simulink model "MPC_Tracking_2020a"  (R2020a)
settings: Solver=VariableStepAuto  StartTime=0.0  StopTime=40  RelTol=1e-3
PostLoadFcn:
  | run('MPC_Tracking_init.m')
  | 
values from neighbouring files (symbols this model uses):
  A = [-1 0; 1 0]    [MPC_Tracking_init.m]
  B = [1;0]    [MPC_Tracking_init.m]
  C = [0,1]    [MPC_Tracking_init.m]
  F = 2*[K_'*Q_*S_; -T_*S_]'    [MPC_Tracking_init.m]
  G = [G;kron(eye(N),-eye(1))]    [MPC_Tracking_init.m]
  H = S_'*Q_*S_ + R_    [MPC_Tracking_init.m]
  N = 10    [MPC_Tracking_init.m]
  S = [zeros(2*N,3)]    [MPC_Tracking_init.m]
  Ts = 1    [MPC_Tracking_init.m]
  W = [delta_umax*ones(N,1);-delta_umin*ones(N,1)]    [MPC_Tracking_init.m]
  x_0 = [8 -5]'    [MPC_Tracking_init.m]
settings Model: Creator=hassan  LastModifiedBy=hassan

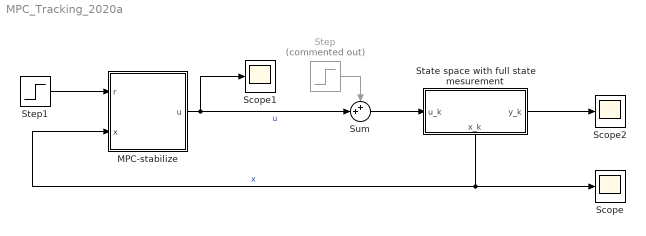
== system MPC_Tracking_2020a ==
  MPC-stabilize : Subsystem
  Scope : Scope
  Scope1 : Scope
  Scope2 : Scope
  State space with full state mesurement : Subsystem
      settings: PortSchema="{\"entries\":[{\"content\":{\"sides\":[{\"content\":{\"connectorIds\":[\"In1\"]},\"type\":\"ConnectorPlacement.EquallySpacedRectSide\",\"uuid\":\"af8233aa-8abb-4886-bf43-cd1df4b87fab\"},{\"content\":{\"connectorIds\":[\"Out1\"],\"side\":\"RIGHT\"},\"type\":\"ConnectorPlacement.EquallySpacedRectSide\",\"uuid\":\"f0184c17-054b-49be-872c-09bd334a5600\"},{\"content\":{\"connectorIds\":[],\"side\":\"TOP\"},\"type\":\"ConnectorPlacement.EquallySpacedRectSide\",\"uuid\":\"196756da-402b-4ddd-adb8-b38ddd7714c4\"},{\"content\":{\"connectorIds\":[\"Out2\"],\"side\":\"BOTTOM\"},\"type\":\"ConnectorPlacement.EquallySpacedRectSide\",\"uuid\":\"e01ecabc-bb09-404c-a3dc-123317d894ec\"}]},\"type\":\"ConnectorPlacement.EquallySpacedConnector\",\"uuid\":\"975ee949-398e-43e2-80ac-c4948e7e5efa\"}],\"packageUris\":[\"http://schema.mathworks.com/mf0/Connector/19700101\"],\"version\":\"1.0\"}"
  Step : Step  Commented=on  Time=20  After=2  SampleTime=0
  Step1 : Step  Time=10  After=6  SampleTime=0
  Sum : Sum  Inputs=++|
  wires:
  State space with full state mesurement/2(x_k) -> MPC-stabilize/2(x), Scope/1  "x"
  MPC-stabilize/1(u) -> Sum/2, Scope1/1  "u"
  State space with full state mesurement/1(y_k) -> Scope2/1
  Sum/1 -> State space with full state mesurement/1(u_k)
  Step/1 -> Sum/1
  Step1/1 -> MPC-stabilize/1(r)

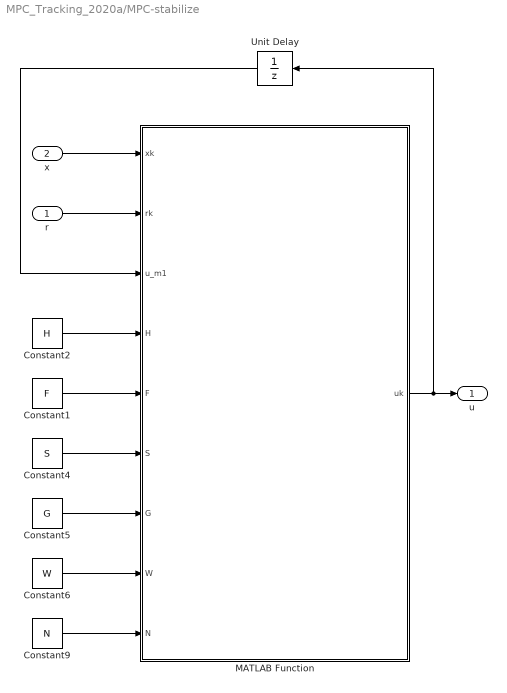
== system MPC_Tracking_2020a/MPC-stabilize ==
  r : Inport
  x : Inport  Port=2
  Constant1 : Constant  Value=F
  Constant2 : Constant  Value=H
  Constant4 : Constant  Value=S
  Constant5 : Constant  Value=G
  Constant6 : Constant  Value=W
  Constant9 : Constant  Value=N
  MATLAB Function : MATLAB Function  TreatAsAtomicUnit=on
  Unit Delay : UnitDelay  SampleTime=Ts  HasFrameUpgradeWarning=on
  u : Outport  VectorParamsAs1DForOutWhenUnconnected=off
  wires:
  x/1 -> MATLAB Function/1(xk)
  Constant2/1 -> MATLAB Function/4(H)
  Constant1/1 -> MATLAB Function/5(F)
  Constant4/1 -> MATLAB Function/6(S)
  Constant5/1 -> MATLAB Function/7(G)
  Constant6/1 -> MATLAB Function/8(W)
  Constant9/1 -> MATLAB Function/9(N)
  MATLAB Function/1(uk) -> u/1, Unit Delay/1
  r/1 -> MATLAB Function/2(rk)
  Unit Delay/1 -> MATLAB Function/3(u_m1)

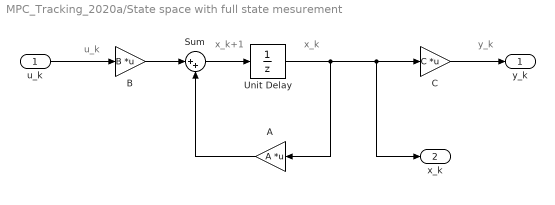
== system MPC_Tracking_2020a/State space with full state mesurement ==
  note: x_k
  note: u_k
  note: x_k+1
  note: y_k
  u_k : Inport
  A : Gain  Gain=A  Multiplication=Matrix(K*u)
  B : Gain  Gain=B  Multiplication=Matrix(K*u)
  C : Gain  Gain=C  Multiplication=Matrix(K*u)
  Sum : Sum  Inputs=|++
  Unit Delay : UnitDelay  InitialCondition=x_0  SampleTime=Ts  HasFrameUpgradeWarning=on
  y_k : Outport  VectorParamsAs1DForOutWhenUnconnected=off
  x_k : Outport  Port=2  VectorParamsAs1DForOutWhenUnconnected=off
  wires:
  B/1 -> Sum/1
  A/1 -> Sum/2
  Sum/1 -> Unit Delay/1
  C/1 -> y_k/1
  u_k/1 -> B/1
  Unit Delay/1 -> A/1, x_k/1, C/1

== matlab function MPC_Tracking_2020a/MPC-stabilize/MATLAB Function ==
  settings: updateMethod=DISCRETE  sampleTime=Ts
  data: xk input; rk input; u_m1 input; uk output; H input; F input; S input; G input; W input; N input
function uk = MPC_Stabilisation(xk,rk,u_m1,H,F,S,G,W,N)

    %m  
     
    coder.extrinsic('optimoptions');
    coder.extrinsic('try');
    options = optimoptions('quadprog');
    options = optimoptions(options, 'Display', 'off');
    coder.extrinsic('quadprog');
    
    %Z = zeros( );

    %sol = quadprog( , , , , [], [], [], [], [], options);  
    
    if ~isempty(sol)
        Z = sol;
    else 
        error('QP Solver: QP problem infeasable, try relaxing constraints.');
    end

    %uk 
      
end
